simulink library "Lib_CerebusRead"  (R2012b)
settings: Solver=ode45  StartTime=0.0  StopTime=10.0  RelTol=1e-3
undefined symbols (not defined in the file): dfilt
libraries: xpcnetworkbufferlib x3, xpcethernetlib x1, xpclib x1, dsparch4 x1, simulink x1
settings Model: Creator=gilja  LastModifiedBy=NPTL

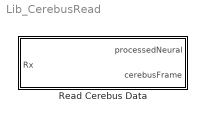
== system Lib_CerebusRead ==
  Read Cerebus Data : Subsystem

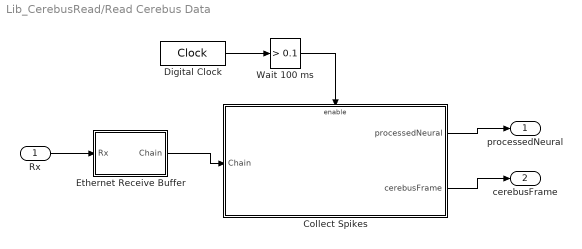
== system Lib_CerebusRead/Read Cerebus Data ==
  Rx : Inport
  Collect Spikes : Subsystem
  Digital Clock : DigitalClock  SampleTime=0.001
  Ethernet Receive Buffer : Subsystem
  Wait 100 ms : simulink/Logic and Bit Operations/Compare To Constant  relop=>  const=0.1  OutDataTypeStr=boolean
  processedNeural : Outport  OutDataTypeStr=Bus: processedNeural
  cerebusFrame : Outport  Port=2  OutDataTypeStr=int16
  wires:
  Rx/1 -> Ethernet Receive Buffer/1(Rx)
  Ethernet Receive Buffer/1(Chain) -> Collect Spikes/1(Chain)
  Digital Clock/1 -> Wait 100 ms/1
  Wait 100 ms/1 -> Collect Spikes/Enable
  Collect Spikes/1(processedNeural) -> processedNeural/1
  Collect Spikes/2(cerebusFrame) -> cerebusFrame/1

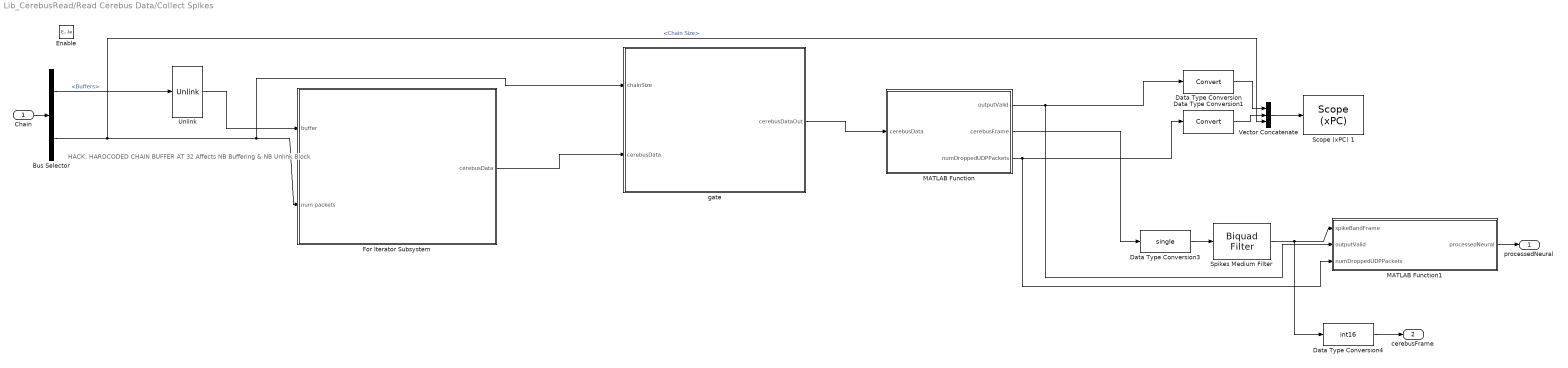
== system Lib_CerebusRead/Read Cerebus Data/Collect Spikes ==
  note: HACK: HARDCODED CHAIN BUFFER AT 32
      | Affects NB Buffering & NB Unlink Block
  Chain : Inport
  Enable : EnablePort  StatesWhenEnabling=reset  PropagateVarSize=During execution
  Bus Selector : BusSelector  OutputSignals=Buffers,Chain Size
  Data Type Conversion : DataTypeConversion
  Data Type Conversion1 : DataTypeConversion
  Data Type Conversion3 : DataTypeConversion  OutDataTypeStr=single
  Data Type Conversion4 : DataTypeConversion  OutDataTypeStr=int16  RndMeth=Nearest
  For Iterator Subsystem : Subsystem  TreatAsAtomicUnit=on
  MATLAB Function : MATLAB Function  TreatAsAtomicUnit=on
  MATLAB Function1 : MATLAB Function  TreatAsAtomicUnit=on
  Scope (xPC) 1 : xpclib/Misc./Scope (xPC)   scopeno=33  scopetype=Target  autostart=on  viewmode=Numerical  formatstr='%15.6f'  grid=on  ylimits=[0,0]  nosamples=250  noprepostsamples=0  interleave=1  triggermode=FreeRun  triggersignal=1  triggerlevel=0.0  triggerslope=Either  triggerscope=1  triggersample=0  filename=data.dat  mode=Lazy  writesize=512  autorestart=off  dynamicfilemode=off  maxwritefilesize=512*1024^2
  Spikes Medium Filter : dsparch4/Biquad Filter  IIRFiltStruct=Direct form II transposed  CoeffSource=Specify via dialog  BiQuadCoeffs="[0.95321773445431  -1.90644870937033 0.95323097500802 1 -1.90514144409761 0.90775595733389;  0.97970016700443  -1.95938672569874 0.97968655878878 1 -1.95804317832840 0.96073029104793]"  a0Flag=Warning  IC=0  ICnum=0  ICden=0  InputProcessing=Columns as channels (frame based)  denAccumFracLength=30  denProdOutputFracLength=30  secondMemoryFracLength=15  roundingMode=Floor  overflowMode=off  ScaleValues=1  optimizeScaleValues=on  ScaleValueMode=Specify via input port (g)  scaleValueFracLength=14  FilterSource=Specify via dialog  dfiltObjectName=dfilt.df2tsos([1 0.3 0.4],[1 0.1 0.2])
  "Unlink " : xpcnetworkbufferlib/Unlink   VectorLength=32
  Vector Concatenate : Concatenate  NumInputs=3
  gate : MATLAB Function  TreatAsAtomicUnit=on
  processedNeural : Outport  OutDataTypeStr=Bus: processedNeural
  cerebusFrame : Outport  Port=2  OutDataTypeStr=int16
  wires:
  Chain/1 -> Bus Selector/1
  Bus Selector/1 -> "Unlink "/1  "<Buffers>"
  "Unlink "/1 -> For Iterator Subsystem/1(buffer)
  Bus Selector/2 -> Vector Concatenate/3, For Iterator Subsystem/2(num packets), gate/1(chainSize)  "<Chain Size>"
  For Iterator Subsystem/1(cerebusData) -> gate/2(cerebusData)
  MATLAB Function/2(cerebusFrame) -> Data Type Conversion3/1
  MATLAB Function/1(outputValid) -> MATLAB Function1/2(outputValid), Data Type Conversion/1
  MATLAB Function/3(numDroppedUDPPackets) -> MATLAB Function1/3(numDroppedUDPPackets), Data Type Conversion1/1
  Data Type Conversion1/1 -> Vector Concatenate/2
  Data Type Conversion/1 -> Vector Concatenate/1
  Vector Concatenate/1 -> Scope (xPC) 1/1
  gate/1(cerebusDataOut) -> MATLAB Function/1(cerebusData)
  Spikes Medium Filter/1 -> Data Type Conversion4/1, MATLAB Function1/1(spikeBandFrame)
  Data Type Conversion3/1 -> Spikes Medium Filter/1
  MATLAB Function1/1(processedNeural) -> processedNeural/1
  Data Type Conversion4/1 -> cerebusFrame/1

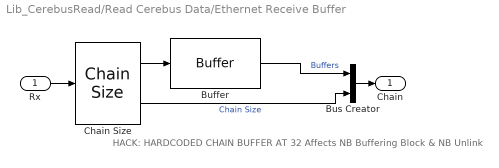
== system Lib_CerebusRead/Read Cerebus Data/Ethernet Receive Buffer ==
  note: HACK: HARDCODED CHAIN BUFFER AT 32
      | Affects NB Buffering Block & NB Unlink
  Rx : Inport
  Buffer : xpcnetworkbufferlib/Buffer   ChainSize=32  BufferSize=0  Threshold=0
  Bus Creator : BusCreator  Inputs=2
  "Chain Size " : xpcnetworkbufferlib/Chain Size 
  Chain : Outport
  wires:
  Buffer/1 -> Bus Creator/1  "Buffers"
  Bus Creator/1 -> Chain/1
  "Chain Size "/2 -> Bus Creator/2  "Chain Size"
  Rx/1 -> "Chain Size "/1
  "Chain Size "/1 -> Buffer/1

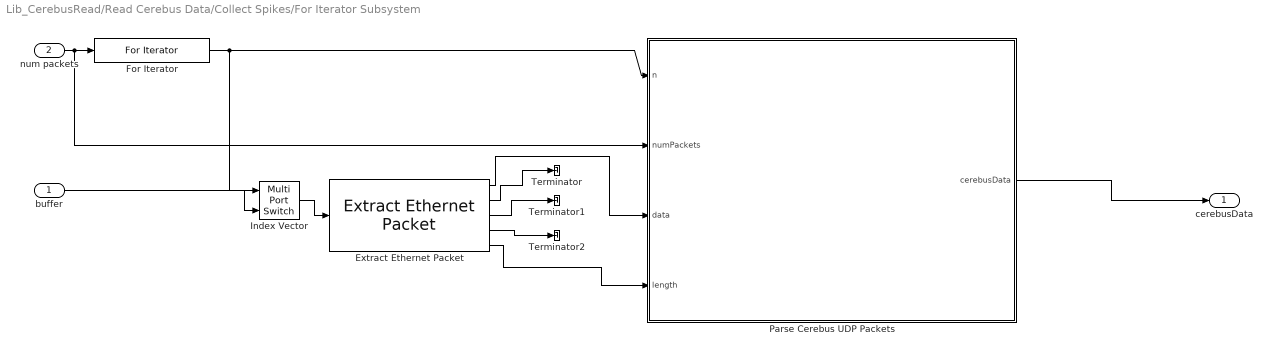
== system Lib_CerebusRead/Read Cerebus Data/Collect Spikes/For Iterator Subsystem ==
  buffer : Inport
  num packets : Inport  Port=2
  Extract Ethernet Packet : xpcethernetlib/Extract Ethernet Packet   EthernetDataSize=1500
  For Iterator : ForIterator  IterationSource=external  IterationVariableDataType=int8
  Index Vector : MultiPortSwitch  Inputs=1
  Parse Cerebus UDP Packets : MATLAB Function  TreatAsAtomicUnit=on
  Terminator : Terminator
  Terminator1 : Terminator
  Terminator2 : Terminator
  cerebusData : Outport  OutDataTypeStr=Bus: cerebusData
  wires:
  For Iterator/1 -> Index Vector/1, Parse Cerebus UDP Packets/1(n)
  Extract Ethernet Packet/5 -> Parse Cerebus UDP Packets/4(length)
  num packets/1 -> For Iterator/1, Parse Cerebus UDP Packets/2(numPackets)
  buffer/1 -> Index Vector/2
  Index Vector/1 -> Extract Ethernet Packet/1
  Extract Ethernet Packet/1 -> Parse Cerebus UDP Packets/3(data)
  Parse Cerebus UDP Packets/1(cerebusData) -> cerebusData/1
  Extract Ethernet Packet/2 -> Terminator/1
  Extract Ethernet Packet/3 -> Terminator1/1
  Extract Ethernet Packet/4 -> Terminator2/1

== matlab function Lib_CerebusRead/Read Cerebus Data/Collect Spikes/For Iterator Subsystem/Parse Cerebus UDP Packets ==
  data: n input; numPackets input; data input; cerebusData output Bus: cerebusData; length input; modelConstants parameter
function cerebusData = parseBroadbandFromCerebus(n, numPackets, data, length, modelConstants)
%#codegen 

%%%%%%%%%%%%%%%%%%%%%%%%%%%%%
%
% parse cerebus broadband with common average referencing
%
% Vikash
% Stanford NPTL
% 2/2012
%
%%%%%%%%%%%%%%%%%%%%%%%%%%%%%



%%%%%%%%%%%%%%%%%%%%%%%%%%%%%
% Generic cbPKT data format
%
% values are little endian
%
% uint32 time  // cerebus 30kHz clock
% uint16 chid  // channel id (must be < 0x8000)
% uint8  type
% uint8  dlen  // number of 32-bit (4 byte) data chunks that follows
% *****  data
%%%%%%%%%%%%%%%%%%%%%%%%%%%%%

%%%%%%%%%%%%%%%%%%%%%%%%%%%%%
% cbPKT spike data format
%
% header info: 20 bytes
% spike waveform, max of 128 points (256 bytes)
% internal lab convention of 48 points (96 bytes) results in 1.2 ms data snippet
%
% uint32 time        // cerebus 30kHz clock
% uint16 chid        // channel id (must be 0 < chid < 145)
% uint8  unit        // unit classification (1-5 = sorted unit num, 0 = unclassified, 31 = artifact, 30 = background)
% uint8  dlen        // length of 32-bit (4 byte) data chunks that follows (fixed to 27 for our lab)
% float  fPattern[2] // used for automatic spike sorting
% int16  nPeak       // highest value in spike
% int16  nValley     // lowest values in spike
% int16  wave[48]    // spike waveform
%%%%%%%%%%%%%%%%%%%%%%%%%%%%%



% constants
numCerebusChannels = modelConstants.cerebus.numCerebusChannels;
cerebusIpSource = modelConstants.cerebus.cerebusIpSource;
cerebusIpDest = modelConstants.cerebus.cerebusIpDest;
maxSamplesInMS = modelConstants.cerebus.maxSamplesInMS;

IP_UDP_HEADER_SIZE = uint16(28); % IP header = 20, UDP header = 8

cbPKT_sample_dlen = uint8(numCerebusChannels/2);   

% static variables
% these will contain the final output variables at the end of the for iterator
persistent samplesP;
persistent sampleTimesP;
persistent numSamplesP;

persistent droppedUDPPacketsP;
persistent lastUDPPacketNumberP;

persistent firstCerebusTimeP;
persistent lastCerebusTimeP;

% init persistents
if isempty(droppedUDPPacketsP)
    samplesP = int16(zeros(maxSamplesInMS, numCerebusChannels));
    sampleTimesP = uint32(zeros(maxSamplesInMS,1));
    numSamplesP = uint32(0);
    
    droppedUDPPacketsP = uint32(0);
    lastUDPPacketNumberP = int32(-1);
    
    firstCerebusTimeP = uint32(0);
    lastCerebusTimeP = uint32(0);
end


if n == 1
    samplesP = int16(zeros(maxSamplesInMS, numCerebusChannels));
    numSamplesP = uint32(0);
    sampleTimesP =uint32(zeros(maxSamplesInMS, 1));
end

% Only process packet if it is from cerebus
if(all(data(13:16) == cerebusIpSource') ...
        && all(data(17:20) == cerebusIpDest'))
    
    % yank current packet num in IP header
    udpPacketNumber = int32(data(5))*int32(256) + int32(data(6));
    
    % check for dropped packet
    if(lastUDPPacketNumberP ~= -1)
        droppedUDPPacketsP = droppedUDPPacketsP + uint32(mod(udpPacketNumber-lastUDPPacketNumberP, 2^16) - 1);
    end
    
    lastUDPPacketNumberP = udpPacketNumber;
    
    cbPKT_startpos = uint16(IP_UDP_HEADER_SIZE+1);
    
    firstCbPkt = true;
        
    % parse and copy each spike cbPKT
    while cbPKT_startpos < length
        
        cbPKT_chid_lsb = data(cbPKT_startpos + 4);  % extract channel lsb
        cbPKT_chid_msb = data(cbPKT_startpos + 5);  % extract channel msb
        cbPKT_type = data(cbPKT_startpos + 6);      % extract unit classification
        cbPKT_dlen = data(cbPKT_startpos + 7);      % extract data length of "non header" data
        
        if( (n== 1) && (firstCbPkt) )
            firstCerebusTimeP = uint32(data(cbPKT_startpos))*2^(0*8) + uint32(data(cbPKT_startpos+1))*2^(1*8) + uint32(data(cbPKT_startpos+2))*2^(2*8) + uint32(data(cbPKT_startpos+3))*2^(3*8);
            firstCbPkt = false;
        end
        
        lastCerebusTimeP = uint32(data(cbPKT_startpos))*2^(0*8) + uint32(data(cbPKT_startpos+1))*2^(1*8) + uint32(data(cbPKT_startpos+2))*2^(2*8) + uint32(data(cbPKT_startpos+3))*2^(3*8);
        
        
        % Check for group packet type 5 (broadband, 30 kS/s)    
        if (cbPKT_chid_lsb == 0) && (cbPKT_chid_msb == 0) && ...
                (cbPKT_dlen == cbPKT_sample_dlen) && ...
                (cbPKT_type == 5)
            
            numSamplesP = numSamplesP + 1;
            
            sampleTimesP(numSamplesP) = uint32(data(cbPKT_startpos))*2^(0*8) + uint32(data(cbPKT_startpos+1))*2^(1*8) + uint32(data(cbPKT_startpos+2))*2^(2*8) + uint32(data(cbPKT_startpos+3))*2^(3*8);
            
            for x = coder.unroll(1:numCerebusChannels)
                tmpSample = int32(data(cbPKT_startpos + 8 + 2*x - 2))*(2^(0*8)) + int32(data(cbPKT_startpos + 8 + 2*x - 1))*(2^(1*8));
                if(tmpSample > 2^15)
                    samplesP(numSamplesP, x) = int16(tmpSample - 2^16);
                else
                    samplesP(numSamplesP, x) = int16(tmpSample);
                end
                
            end
            % Common average reference:
            samplesP(numSamplesP, :) = samplesP(numSamplesP, :) - mean(samplesP(numSamplesP, :)); 
        end
        
        cbPKT_startpos = cbPKT_startpos + uint16(8) + uint16(cbPKT_dlen)*4;
    end
    
    
end

cerebusData.droppedUDPPackets = droppedUDPPacketsP;
cerebusData.lastUDPPacketNumber = lastUDPPacketNumberP;

% update large arrays only at end of for loop
if n == numPackets
    cerebusData.numSamples = numSamplesP;
    cerebusData.samples = samplesP;
    cerebusData.sampleTimes = sampleTimesP;
    
    cerebusData.firstCerebusTime = firstCerebusTimeP;
    cerebusData.lastCerebusTime = lastCerebusTimeP;
else
    cerebusData.numSamples = uint32(0);
    cerebusData.samples = coder.nullcopy(int16(zeros(maxSamplesInMS, numCerebusChannels)));
    cerebusData.sampleTimes = coder.nullcopy(uint32(zeros(maxSamplesInMS,1)));
    
    cerebusData.firstCerebusTime = uint32(0);
    cerebusData.lastCerebusTime = uint32(0);
end

== matlab function Lib_CerebusRead/Read Cerebus Data/Collect Spikes/MATLAB Function1 ==
  data: spikeBandFrame input; outputValid input; numDroppedUDPPackets input; modelConstants parameter; processedNeural output Bus: processedNeural
function processedNeural = extractNerualMaxMin(spikeBandFrame, outputValid, numDroppedUDPPackets, modelConstants)
%#codegen
persistent bufferMeanSquared bufferIdx bufferCnt bufferReady;

if(isempty(bufferCnt))
    bufferCnt = 0;
    bufferIdx = 0;
    bufferMeanSquared = single(zeros(2, size(spikeBandFrame, 2)));
    bufferReady = false;
end

if (bufferCnt == modelConstants.RMSperiod)
    bufferIdx = 1 - bufferIdx;
    bufferMeanSquared(2-bufferIdx, :) = 0;
    bufferCnt = 0;
    bufferReady = true;
end

bufferMeanSquared(2-bufferIdx, :) = bufferMeanSquared(2-bufferIdx, :) + mean(spikeBandFrame.^2) / modelConstants.RMSperiod; 
bufferCnt = bufferCnt + 1;

if(bufferReady && (bufferCnt <= size(spikeBandFrame, 2)))
    processedNeural.meanSquared = bufferMeanSquared(bufferIdx + 1, bufferCnt);
    processedNeural.meanSquaredChannel = uint8(bufferCnt);
else
    processedNeural.meanSquared = single(0);
    processedNeural.meanSquaredChannel = uint8(0);
end
   
   
[processedNeural.minSpikeBand tmpMin] = min(spikeBandFrame);
processedNeural.minSpikeBandInd = uint8(tmpMin);
[processedNeural.maxSpikeBand tmpMax] = max(spikeBandFrame);
processedNeural.maxSpikeBandInd = uint8(tmpMax);
processedNeural.outputValid = outputValid;
processedNeural.numDroppedUDPPackets = numDroppedUDPPackets;

== matlab function Lib_CerebusRead/Read Cerebus Data/Collect Spikes/MATLAB Function ==
  data: cerebusData input Bus: cerebusData; outputValid output boolean size=1; modelConstants parameter; cerebusFrame output int16 size=[30 modelConstants.cerebus.numCerebusChannels]; numDroppedUDPPackets output
function [outputValid, cerebusFrame, numDroppedUDPPackets] = bufferCerebusSamples(cerebusData, modelConstants)
%#codegen

persistent sampleBuffer bufferInIdx bufferOutIdx outputValidP bufferInit;

numCerebusChannels = modelConstants.cerebus.numCerebusChannels;
bufferSize = modelConstants.cerebus.sampleBufferSize;
bufferDelay = modelConstants.cerebus.sampleBufferDelay;


if(isempty(sampleBuffer))
    sampleBuffer = int16(zeros(bufferSize, numCerebusChannels));
    bufferInIdx = 0;
    bufferOutIdx = bufferSize;
    outputValidP = false;
    bufferInit = true;
end

cerebusFrame = int16(zeros(30, numCerebusChannels));

if(bufferInIdx < bufferOutIdx)
    bufferSpace = bufferOutIdx - bufferInIdx;
else
    bufferSpace = bufferSize - bufferInIdx + bufferOutIdx;
end

if(cerebusData.numSamples > bufferSpace)
    bufferInit = false;
    outputValidP = false;
end

if((cerebusData.numSamples > 0) && (cerebusData.numSamples < bufferSize))
    sampleBuffer(bufferInIdx + [1:cerebusData.numSamples], :) = cerebusData.samples(1:cerebusData.numSamples, :);
    bufferInIdx = mod((bufferInIdx + double(cerebusData.numSamples)), bufferSize);
end

if(bufferInit)
    if(bufferInIdx >= (bufferDelay))
        bufferInit = false;
        outputValidP = true;
    end
elseif(outputValidP)
    numToEndOfBuffer = bufferSize - bufferOutIdx;
    if( (numToEndOfBuffer >= 30) && ...
            ((bufferInIdx >= bufferOutIdx + 30) || (bufferInIdx < bufferOutIdx)) )
        cerebusFrame = sampleBuffer(bufferOutIdx+[1:30], :);
        
    elseif ( (numToEndOfBuffer < 30) ...
            && (bufferInIdx >= (30 - numToEndOfBuffer) ))
        idx = [1:30];
        idx(1:numToEndOfBuffer) = idx(1:numToEndOfBuffer) + bufferOutIdx;
        idx(numToEndOfBuffer+1:end) = idx(numToEndOfBuffer+1:end) - numToEndOfBuffer;
        cerebusFrame = sampleBuffer(idx, :);
        
    else
        outputValidP = false;
    end
    
    bufferOutIdx = mod((bufferOutIdx + 30), bufferSize);
end


outputValid = outputValidP;
numDroppedUDPPackets = cerebusData.droppedUDPPackets;

== matlab function Lib_CerebusRead/Read Cerebus Data/Collect Spikes/gate ==
  data: chainSize input; cerebusDataOut output Bus: cerebusData; cerebusData input Bus: cerebusData; modelConstants parameter
function cerebusDataOut = checkNoPackets(chainSize, cerebusData, modelConstants)


if chainSize == 0
    cerebusData.samples = coder.nullcopy(int16(zeros(modelConstants.cerebus.maxSamplesInMS, modelConstants.cerebus.numCerebusChannels)));
    cerebusData.sampleTimes = coder.nullcopy(uint32(zeros(modelConstants.cerebus.maxSamplesInMS,1)));
    cerebusData.numSamples = uint32(0);
    
    cerebusData.firstCerebusTime = uint32(0);
    cerebusData.lastCerebusTime = uint32(0);
end

cerebusDataOut = cerebusData;
